simulink model "GLO_tracking_model_no_ptu_dynamics"  (R2016a)
settings: Solver=VariableStepAuto  StartTime=0.0  StopTime=40  MaxStep=0.01  RelTol=1e-4
libraries: simulink x1
settings Model: Creator=addiewan  LastModifiedBy=addiewan
settings DataIOCC: LimitDataPoints=on  SaveOutput=off  SaveTime=off
settings OptimizationCC: ExpressionDepthLimit=2147483647  LifeSpan=1
settings DebuggingCC: UnderspecifiedInitializationDetection=Classic  MergeDetectMultiDrivingBlocksExec=none  FcnCallInpInsideContextMsg=EnableAllAsWarning  AllowSymbolicDim=off  StateNameClashWarn=warning
settings GRTTargetCC: CombineOutputUpdateFcns=off  GRTInterface=on

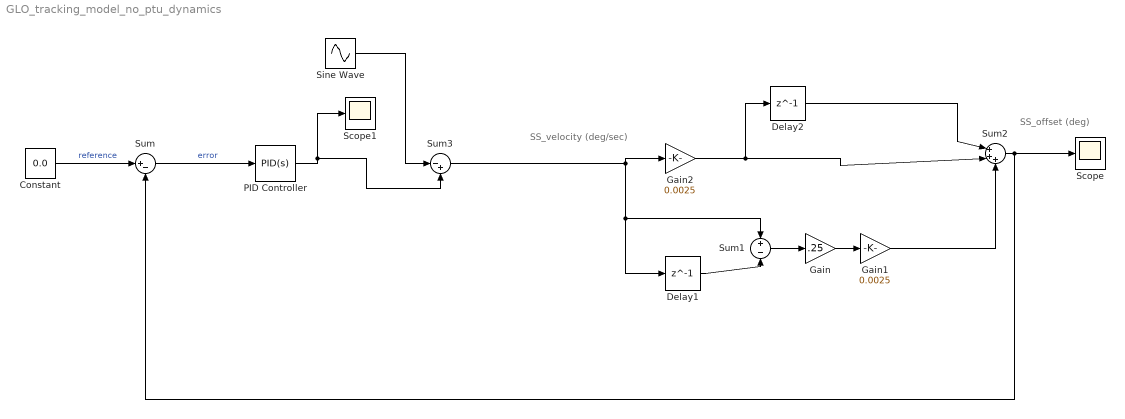
== system GLO_tracking_model_no_ptu_dynamics ==
  note: SS_velocity (deg/sec)
  note: SS_offset (deg)
  Constant : Constant  Value=0.0
  Delay1 : Delay  DelayLength=1  InitialCondition=0
  Delay2 : Delay  DelayLength=1  InitialCondition=0
  Gain : Gain  Gain=.25
  Gain1 : Gain  Gain=0.0025
  Gain2 : Gain  Gain=0.0025
  PID Controller : simulink/Continuous/PID Controller  Controller=PID  TimeDomain=Continuous-time  SampleTime=-1  IntegratorMethod=Forward Euler  FilterMethod=Forward Euler  Form=Parallel  UseFilter=on  ControllerParametersSource=internal  P=1  I=1  D=0  N=100  InitialConditionSource=internal  InitialConditionForIntegrator=0  InitialConditionForFilter=0  ExternalReset=none  LimitOutput=off  UpperSaturationLimit=inf  LowerSaturationLimit=-inf  LinearizeAsGain=on  AntiWindupMode=none  Kb=1  TrackingMode=off  Kt=1  PParamMin=[]  PParamMax=[]  IParamMin=[]  IParamMax=[]  DParamMin=[]  DParamMax=[]  NParamMin=[]  NParamMax=[]  KbParamMin=[]  KbParamMax=[]  KtParamMin=[]  KtParamMax=[]  POutMin=[]  POutMax=[]  IOutMin=[]  IOutMax=[]  DOutMin=[]  DOutMax=[]  NOutMin=[]  NOutMax=[]  KbOutMin=[]  KbOutMax=[]  KtOutMin=[]  KtOutMax=[]  IntegratorOutMin=[]  IntegratorOutMax=[]  FilterOutMin=[]  FilterOutMax=[]  SumOutMin=[]  SumOutMax=[]  SumI1OutMin=[]  SumI1OutMax=[]  SumI2OutMin=[]  SumI2OutMax=[]  SumI3OutMin=[]  SumI3OutMax=[]  SumDOutMin=[]  SumDOutMax=[]  SaturationOutMin=[]  SaturationOutMax=[]  IntegratorContinuousStateAttributes=''  IntegratorStateMustResolveToSignalObject=off  IntegratorRTWStateStorageClass=Auto  FilterContinuousStateAttributes=''  FilterStateMustResolveToSignalObject=off  FilterRTWStateStorageClass=Auto  DifferentiatorICPrevScaledInput=0  DifferentiatorOutMin=[]  DifferentiatorOutMax=[]
  Scope : Scope
  Scope1 : Scope
  Sine Wave : Sin  Frequency=.1  SampleTime=1/10
  Sum : Sum  Inputs=|+-
  Sum1 : Sum  Inputs=+-
  Sum2 : Sum  Inputs=|+++
  Sum3 : Sum  Inputs=|-+
  wires:
  Constant/1 -> Sum/1  "reference"
  Delay1/1 -> Sum1/2
  Sum1/1 -> Gain/1
  Gain/1 -> Gain1/1
  Gain1/1 -> Sum2/3
  Delay2/1 -> Sum2/1
  Sum2/1 -> Scope/1, Sum/2
  Sine Wave/1 -> Sum3/1
  Sum3/1 -> Gain2/1, Sum1/1, Delay1/1
  Gain2/1 -> Delay2/1, Sum2/2
  Sum/1 -> PID Controller/1  "error"
  PID Controller/1 -> Scope1/1, Sum3/2
